simulink model "BCM2_4"  (R2021b)
settings: Solver=FixedStepDiscrete  StartTime=0.0  StopTime=1  FixedStep=0.001  RelTol=1e-3  EnableMultiTasking=on
InitFcn:
  | mbd_mpc_consistency_checks(bdroot(gcs));
model workspace (MAT data in the model file):
  CAN_rec : Simulink.Signal (value not decoded)
  CAN_transm_stat : Simulink.Signal (value not decoded)
  CAN_trm : Simulink.Signal (value not decoded)
  DITHER_CFB0 : Simulink.Parameter (value not decoded)
  DITHER_CFB1 : Simulink.Parameter (value not decoded)
  DITHER_CFB2 : Simulink.Parameter (value not decoded)
  DITHER_EN0 : Simulink.Parameter (value not decoded)
  DITHER_EN1 : Simulink.Parameter (value not decoded)
  DITHER_EN2 : Simulink.Parameter (value not decoded)
  DITHER_SIZE0 : Simulink.Parameter (value not decoded)
  DITHER_SIZE1 : Simulink.Parameter (value not decoded)
  DITHER_SIZE2 : Simulink.Parameter (value not decoded)
  DITHER_STEP0 : Simulink.Parameter (value not decoded)
  DITHER_STEP1 : Simulink.Parameter (value not decoded)
  DITHER_STEP2 : Simulink.Parameter (value not decoded)
  DITHER_SYNC0 : Simulink.Parameter (value not decoded)
  DITHER_SYNC1 : Simulink.Parameter (value not decoded)
  DITHER_SYNC2 : Simulink.Parameter (value not decoded)
  ECUMbut : Simulink.Signal (value not decoded)
  FAULTN : Simulink.Signal (value not decoded)
  FM0 : Simulink.Parameter (value not decoded)
  FM1 : Simulink.Parameter (value not decoded)
  FM2 : Simulink.Parameter (value not decoded)
  FME : Simulink.Parameter (value not decoded)
  Fsys_M : Simulink.Parameter (value not decoded)
  Fsys_N : Simulink.Parameter (value not decoded)
  Fsys_WDEN : Simulink.Parameter (value not decoded)
  Fsys_div : Simulink.Parameter (value not decoded)
  HL0 : Simulink.Parameter (value not decoded)
  HL1 : Simulink.Parameter (value not decoded)
  HL2 : Simulink.Parameter (value not decoded)
  IDIAG0 : Simulink.Parameter (value not decoded)
  IDIAG1 : Simulink.Parameter (value not decoded)
  IDIAG2 : Simulink.Parameter (value not decoded)
  Ivalve : Simulink.Signal (value not decoded)
  KI_index0 : Simulink.Parameter (value not decoded)
  KI_index1 : Simulink.Parameter (value not decoded)
  KI_index2 : Simulink.Parameter (value not decoded)
  PWM_Period0 : Simulink.Parameter (value not decoded)
  PWM_Period1 : Simulink.Parameter (value not decoded)
  PWM_Period2 : Simulink.Parameter (value not decoded)
  RESN : Simulink.Signal (value not decoded)
  SR0 : Simulink.Parameter (value not decoded)
  SR1 : Simulink.Parameter (value not decoded)
  SR2 : Simulink.Parameter (value not decoded)
  Vparam : Simulink.Signal (value not decoded)
  block_tle : Simulink.Signal (value not decoded)
  disp : Simulink.Signal (value not decoded)
  ee_adr : Simulink.Signal (value not decoded)
  ee_en_rd : Simulink.Signal (value not decoded)
  ee_en_wr : Simulink.Signal (value not decoded)
  ee_idle : Simulink.Signal (value not decoded)
  ee_read : Simulink.Signal (value not decoded)
  ee_recv : Simulink.Signal (value not decoded)
  ee_send : Simulink.Signal (value not decoded)
  in_stats : Simulink.Signal (value not decoded)
  inputs : Simulink.Signal (value not decoded)
  light : Simulink.Signal (value not decoded)
  out_drv : Simulink.Signal (value not decoded)
  out_drv_test : Simulink.Signal (value not decoded)
  out_test_en : Simulink.Signal (value not decoded)
  recv_spi2 : Simulink.Signal (value not decoded)
  ret : Simulink.Signal (value not decoded)
  spi_rcv_tle82453 : Simulink.Signal (value not decoded)
  tle82453_Ivlv : Simulink.Signal (value not decoded)
  tle82453_err : Simulink.Signal (value not decoded)
  tle82453_reset : Simulink.Signal (value not decoded)
  wtdg_CAN : Simulink.Signal (value not decoded)
symbols that are objects in the model workspace (value not decoded): CAN_rec, CAN_transm_stat, ECUMbut, inputs, Ivalve, out_drv_test, recv_spi2, ret, SR0, tle82453_Ivlv
undefined symbols (not defined in the file or in its folder): color, LQFP
libraries: simulink x68, mbd_mpc574x_ec_toolbox x50, canmsglib x42, hdlsllib x9, commutil2 x7, etargetslib x4
(part 6 of 6)

== stateflow chart BCM2_4/ecumaster12 ==
  settings: updateMethod=DISCRETE  sampleTime=0.01
  state scan_buttons [function]
    (default) -> (junction 38)
    (junction 38) -> (junction 40) : {index=1;}
    (junction 40) -> (junction 39) [order 1] : [index<13]
    (junction 39) -> (junction 46) [order 2]
    (junction 46) -> (junction 40) : {index = index + 1}
    (junction 39) -> (junction 44) [order 1] : [~ECUMbut.arr12(index) && trig(index)]{trig(index)=false}
    (junction 40) -> (junction 43) [order 2]
    (junction 44) -> (junction 46)
  state off
    scan_buttons()
    button_work()
  state button_work [function]
    note: Управление доп фарами
    note: Управление габаритами и ближним
    note: Аварийка
    note: Яркость пилота
    note: Check АКП
    note: Вентилятор пилота
    note: Таблицы ДВС
    note: Обогрев лобового стекла
    note: Электросигнал
    note: Подпирающий топливный насос
    note: Страницы -
    note: Страницы +
    note: Моргание аварийкой
    (default) -> (junction 519)
    (junction 519) -> (junction 521) [order 1] : [ECUMbut.arr12(1) && ~trig(1)]{trig(1)=true}
    (junction 521) -> (junction 530) : {light.dop=~light.dop}
    (junction 530) -> (junction 531) [order 1] : [light.dop]{ECUMbut.color12(1) = color.blue}
    (junction 519) -> (junction 599) [order 2]
    (junction 530) -> (junction 520) [order 2] : {ECUMbut.color12(1) = color.off}
    (junction 531) -> (junction 528)
    (junction 520) -> (junction 599)
    (junction 528) -> (junction 520)
    (junction 599) -> (junction 589)
    (junction 589) -> (junction 577) [order 1] : [ECUMbut.arr12(2) && ~trig(2)]{trig(2)=true}
    (junction 577) -> (junction 584) [order 1] : [cnt_light <2]{cnt_light = cnt_light + 1}
    (junction 570) -> (junction 576) [order 1] : [cnt_light==2]{light.light=true;light.beam=true;ECUMbut.color12(2) = color.blue}
    (junction 589) -> (junction 653) [order 2]
    (junction 577) -> (junction 582) [order 2]
    (junction 584) -> (junction 568)
    (junction 576) -> (junction 579)
    (junction 582) -> (junction 568) : {cnt_light=0}
    (junction 568) -> (junction 570)
    (junction 570) -> (junction 579) [order 2] : [cnt_light==1]{light.light=true;light.beam=false;ECUMbut.color12(2) = color.green}
    (junction 570) -> (junction 575) [order 3] : {light.light=false;light.beam=false;ECUMbut.color12(2) = color.off}
    (junction 579) -> (junction 575)
    (junction 575) -> (junction 653)
    (junction 653) -> (junction 514)
    (junction 514) -> (junction 553) [order 1] : [ECUMbut.arr12(3) && ~trig(3)]{trig(3)=true}
    (junction 553) -> (junction 554) : {ECUMbut.hazard=~ECUMbut.hazard}
    (junction 514) -> (junction 502) [order 2]
    (junction 554) -> (junction 555)
    (junction 555) -> (junction 502)
    (junction 502) -> (junction 516)
    (junction 516) -> (junction 546) [order 1] : [ECUMbut.arr12(4) && ~trig(4)]{trig(4)=true}
    (junction 546) -> (junction 535) : {ECUMbut.bright_pilot=~ECUMbut.bright_pilot}
    (junction 535) -> (junction 539) [order 1] : [ECUMbut.bright_pilot]{ECUMbut.color12(4) = color.bluegreen}
    (junction 516) -> (junction 560) [order 2]
    (junction 535) -> (junction 542) [order 2] : {ECUMbut.color12(4) = color.off}
    (junction 539) -> (junction 540)
    (junction 542) -> (junction 560)
    (junction 540) -> (junction 542)
    (junction 560) -> (junction 504)
    (junction 504) -> (junction 485) [order 1] : [ECUMbut.arr12(5)]{ECUMbut.color12(5) = color.orange}
    (junction 485) -> (junction 490)
    (junction 504) -> (junction 602) [order 2]
    (junction 602) -> (junction 490) [order 1] : [~ECUMbut.arr12(5)]{ECUMbut.color12(5) = color.off}
    (junction 490) -> (junction 475)
    (junction 602) -> (junction 496) [order 2]
    (junction 475) -> (junction 496)
    (junction 496) -> (junction 505)
    (junction 483) -> (junction 487) : {ECUMbut.fan=~ECUMbut.fan}
    (junction 487) -> (junction 489) [order 1] : [ECUMbut.fan]{ECUMbut.color12(6) = color.red}
    (junction 505) -> (junction 483) [order 1] : [ECUMbut.arr12(6) && ~trig(6)]{trig(6)=true}
    (junction 487) -> (junction 471) [order 2] : {ECUMbut.color12(6) = color.off}
    (junction 489) -> (junction 482)
    (junction 505) -> (junction 517) [order 2]
    (junction 471) -> (junction 517)
    (junction 482) -> (junction 471)
    (junction 517) -> (junction 499)
    (junction 499) -> (junction 615) [order 1] : [ECUMbut.arr12(7) && ~trig(7)]{trig(7)=true}
    (junction 615) -> (junction 564) : {ECUMbut.table_rom = ~ECUMbut.table_rom}
    (junction 564) -> (junction 597) [order 1] : [ECUMbut.table_rom]{ECUMbut.color12(7) = color.red}
    (junction 499) -> (junction 491) [order 2]
    (junction 564) -> (junction 592) [order 2] : {ECUMbut.color12(7) = color.off}
    (junction 597) -> (junction 593)
    (junction 592) -> (junction 491)
    (junction 593) -> (junction 592)
    (junction 491) -> (junction 498)
    (junction 498) -> (junction 618) [order 1] : [ECUMbut.arr12(8) && ~trig(8)]{trig(8)=true}
    (junction 618) -> (junction 623) : {ECUMbut.heat=~ECUMbut.heat}
    (junction 623) -> (junction 612) [order 1] : [ECUMbut.heat]{ECUMbut.color12(8) = color.green}
    (junction 498) -> (junction 493) [order 2]
    (junction 623) -> (junction 619) [order 2] : {ECUMbut.color12(8) = color.off}
    (junction 612) -> (junction 613)
    (junction 613) -> (junction 619)
    (junction 619) -> (junction 493)
    (junction 493) -> (junction 466)
    (junction 466) -> (junction 611) [order 1] : [ECUMbut.arr12(9)]{ECUMbut.color12(9) = color.orange}
    (junction 466) -> (junction 660) [order 2]
    (junction 611) -> (junction 617)
    (junction 660) -> (junction 617) [order 1] : [~ECUMbut.arr12(9)]{ECUMbut.color12(9) = color.off}
    (junction 617) -> (junction 610)
    (junction 660) -> (junction 650) [order 2]
    (junction 610) -> (junction 650)
    (junction 650) -> (junction 661)
    (junction 661) -> (junction 629) [order 1] : [ECUMbut.arr12(10) && ~trig(10)]{trig(10)=true}
    (junction 629) -> (junction 563) : {ECUMbut.pump=~ECUMbut.pump}
    (junction 563) -> (junction 608) [order 1] : [ECUMbut.pump]{ECUMbut.color12(10) = color.bluegreen}
    (junction 661) -> (junction 463) [order 2]
    (junction 563) -> (junction 594) [order 2] : {ECUMbut.color12(10) = color.off}
    (junction 608) -> (junction 625)
    (junction 625) -> (junction 594)
    (junction 594) -> (junction 463)
    (junction 463) -> (junction 465)
    (junction 465) -> (junction 621) [order 1] : [ECUMbut.arr12(11)]{ECUMbut.color12(11) = color.white}
    (junction 465) -> (junction 603) [order 2]
    (junction 621) -> (junction 646)
    (junction 603) -> (junction 646) [order 1] : [~ECUMbut.arr12(11)]{ECUMbut.color12(11) = color.off}
    (junction 646) -> (junction 642)
    (junction 603) -> (junction 666) [order 2]
    (junction 642) -> (junction 666)
    (junction 666) -> (junction 664)
    (junction 664) -> (junction 649) [order 1] : [ECUMbut.arr12(12)]{ECUMbut.color12(12) = color.white}
    (junction 664) -> (junction 657) [order 2]
    (junction 649) -> (junction 507)
    (junction 657) -> (junction 507) [order 1] : [~ECUMbut.arr12(12)]{ECUMbut.color12(12) = color.off}
    (junction 657) -> (junction 655) [order 2]
    (junction 507) -> (junction 630)
    (junction 630) -> (junction 655)
    (junction 655) -> (junction 667)
    (junction 667) -> (junction 671) [order 1] : [lamp_hazard]{ECUMbut.color12(3) = color.red}
    (junction 667) -> (junction 675) [order 2]
    (junction 671) -> (junction 678)
    (junction 675) -> (junction 678) [order 1] : [~lamp_hazard]{ECUMbut.color12(3) = color.off}
    (junction 675) -> (junction 684) [order 2]
    (junction 678) -> (junction 682)
    (junction 682) -> (junction 684)
  (default) -> off
  data: trig local boolean size=[1 12] =false; cnt_light local uint8 size=1 =uint8(0); lamp_hazard input boolean size=1; ECUMbut data_store_memory; light data_store_memory

== stateflow chart BCM2_4/поворотники ==
  settings: updateMethod=DISCRETE  sampleTime=0.1
  state blink
    state Delay
      en: i=0
      scan(true)
      du: i = i + 1
    state Delay1
      en: i=0
      scan(false)
      du: i = i + 1
    (default) -> Delay
    Delay1 -> Delay : [i>4]
    Delay -> Delay1 : [i>2]
  state scan(x) [function]
    (default) -> (junction 14)
    (junction 14) -> (junction 26) [order 1] : [left]{outL=x}
    (junction 26) -> (junction 28)
    (junction 14) -> (junction 28) [order 2]
    (junction 28) -> (junction 31) [order 1] : [right]{outR=x}
    (junction 31) -> (junction 33)
    (junction 28) -> (junction 33) [order 2]
    (junction 33) -> (junction 36) [order 1] : [hazard]{outR=x;outL=x;outH=x}
    (junction 36) -> (junction 38)
    (junction 33) -> (junction 38) [order 2]
  state start
    outL=false
    outR = false
    outH = false
  (default) -> start
  start -> blink : [left || right || hazard]
  blink -> start : [~left && ~right && ~hazard]
  data: x function_input; i local uint8 size=1; hazard input boolean size=1; left input boolean size=1; right input boolean size=1; outH output boolean size=1; outL output boolean size=1; outR output boolean size=1

== stateflow chart BCM2_4/CAN1 Transmit buf 27-43/Цвет клавиатуры 12 buf = 28/Цвет клавиатуры buf = 28/Chart ==
  (default) -> (junction 58)
  (junction 58) -> (junction 46) : {temp=0;}
  (junction 46) -> (junction 48) : {i=0;}
  (junction 48) -> (junction 57) [order 2] : {out[0] = (temp & 255);
      |  out[1] = (temp>>8) & 255;
      |  out[2] = (temp>>16)  & 255;
      |  out[3] = (temp>>24)  & 255;}
  (junction 48) -> (junction 47) [order 1] : [i<12]
  (junction 50) -> (junction 48)
  (junction 47) -> (junction 49) : {temp = temp | (input[i] & 1) << (0+i);
      | temp = temp | ((input[i] & 2)>>1) << (12 + i);
      | temp = temp | ((input[i] & 4)>>2) << (24 + i);}
  (junction 49) -> (junction 50) : {i++;}
  data: i local uint8 size=1 =uint8(0); input input uint8 size=12; temp local double size=1; out output uint8 size=8

== stateflow chart BCM2_4/CAN1 Transmit buf 27-43/подсветка клавиатуры buf = 29/подсветка клавиатуры buf = 29/Chart ==
  state backlight_bright
    en:
    out(1) = 0x2F
    out(2) = 3
    out(3) = 0x20
    out(4) = 2
    out(5) = 0x00 % level
  state key_bright1
    en:
    out(1) = 0x2F
    out(2) = 3
    out(3) = 0x20
    out(4) = 1
    out(5) = 0x0F %level
  note: Яркость клавиш при вкл подсветки клавиш
  state backlight_color1
    en:
    out(1) = 0x2F
    out(2) = 3
    out(3) = 0x20
    out(4) = 4
    out(5) = 9
  note: red(1)
      | green(2)
      | blue(3)
      | yellow(4)
      | bluegreen(5)
      | purple(6)
      | white(7)
      | orange(8)
      | yel_green(9)
  state key_bright
    en:
    out(1) = 0x2F
    out(2) = 3
    out(3) = 0x20
    out(4) = 1
    out(5) = 0x30 %level
  state backlight_bright1
    en:
    out(1) = 0x2F
    out(2) = 3
    out(3) = 0x20
    out(4) = 2
    out(5) = 0x04 % level
  note: Яркость подсветки
  note: Яркость клавиш
  (default) -> backlight_bright
  key_bright1 -> backlight_bright : [~ECUMbut.bright_pilot]
  backlight_bright -> key_bright
  backlight_color1 -> key_bright1
  backlight_bright1 -> backlight_color1
  key_bright -> backlight_bright1 : [ECUMbut.bright_pilot]
  data: out output uint8 size=8; ECUMbut data_store_memory

== stateflow chart BCM2_4/retarder ==
  settings: updateMethod=DISCRETE  sampleTime=0.1
  state Diagnostic
    en:
    Ivalve(1)=0
    Ivalve(2)=0
  state work
    state ret_off
      Ivalve(1)=0
      Ivalve(2)=0
    state ret_on
      state ret_on
        ret.M = uint16(ret.stepM(ret.step) * 4000)
        Ivalve(1)=450
      state ret_stdby
        Ivalve(1)=0
        Ivalve(2)=0
      state table
      (default) -> ret_stdby
      ret_stdby -> work.ret_on.ret_on : [Vparam.BrakePos > brk_lvl]
      work.ret_on.ret_on -> ret_stdby [order 1] : [Vparam.BrakePos < (brk_lvl - 2)]
      work.ret_on.ret_on -> table [order 2]
      table -> work.ret_on.ret_on
    state temp_protect
      Ivalve(1)=0
      Ivalve(2)=0
    state diable_pedal
      Ivalve(1)=0
      Ivalve(2)=0
    (default) -> ret_off
    work.ret_on -> ret_off [order 1] : [~ret.ret_en]
    ret_off -> work.ret_on : [ret.ret_en]
    work.ret_on -> temp_protect [order 2] : [ret.RetTemp > 145]
    temp_protect -> work.ret_on : [ret.RetTemp < 120]
    work.ret_on -> diable_pedal [order 3] : [Vparam.PedalPos > 3]
    diable_pedal -> work.ret_on : [Vparam.PedalPos < 1]
  (default) -> Diagnostic
  Diagnostic -> work : [diag == false]
  work -> Diagnostic : [diag == true]
  data: sf_internal_action_state_placeholder_data local double size=1 =0; ret data_store_memory; Vparam data_store_memory; brk_lvl constant uint8 =5; Ivalve data_store_memory; temp_protect output boolean; diable_pedal output boolean; diag input boolean

== stateflow chart BCM2_4/подогрев стекла ==
  settings: updateMethod=DISCRETE  sampleTime=1
  state off
    out = false
  state on
    state on
      en: i=1
      out=true
      du: i = i + 1
    state off
      en: i=1
      out=false
      du: i = i + 1
    (default) -> on.on
    on.off -> on.on : [i>=heat_off * 60]
    on.on -> on.off : [i>=heat_on * 60]
  (default) -> off
  off -> on : [heat]
  on -> off : [~heat]{out=false}
  data: out output boolean size=1; i local; heat input boolean size=1; heat_on parameter; heat_off parameter

== stateflow chart BCM2_4/CAN EEPROM R//W ==
  state ee_wr
    ee_adr = CAN_rec.ee_adr
    ee_send = CAN_rec.ee_data
    % записываем в eeprom
  state x = ee_idl [function]
    (default) -> (junction 28)
    (junction 28) -> (junction 29) [order 1] : [~ee_idle && ~ee_en_rd && ~ee_en_wr]
    (junction 29) -> (junction 31)
    (junction 28) -> (junction 30) [order 2] : {x=true}
    (junction 31) -> (junction 30) : {x = false}
  state ee_idle
    % свободна ли EEPROM?
  state Start
  state ee_idle1
  state ee_idle2
  state ready
    en:
    CAN_trm.ee_adr=CAN_rec.ee_adr;
    CAN_trm.ee_cmd = CAN_rec.ee_cmd;
    CAN_trm.ee_data = ee_read;
    ex: ee_en_rd = false % выключаем чтение из еепром
    CAN_rec.ee_rec_stat = false;
    CAN_trm.ee_en_trm = true;
  state ee_rd
    % запускаем чтение с еепром
  ee_idle -> ee_wr : [~ee_idle && ~ee_en_rd && ~ee_en_wr]{ee_en_wr = true}
  (junction 3) -> ee_idle [order 2] : [CAN_rec.ee_cmd == CMD_WRITE]
  ee_wr -> (junction 66) : [~ee_idle]% ждем окончания записи
      | {ee_en_wr = false}% отключаем запись eeprom
  (default) -> Start
  ee_idle2 -> ee_idle1 [order 2]
  Start -> (junction 3) : [CAN_rec.ee_rec_stat]
  (junction 3) -> ee_idle1 [order 1] : [CAN_rec.ee_cmd == CMD_READ]
  (junction 3) -> (junction 48) [order 3]
  ee_idle1 -> ee_idle2 : [~ee_idl]
      | % ждем готовность еепром
  ee_idle2 -> ee_rd [order 1] : [~ee_idl]{ee_adr = CAN_rec.ee_adr; ee_en_rd = true;}
  (junction 48) -> Start
  ee_rd -> ready : [~ee_idle] % дожидаемся конца чтения
  ready -> Start
  (junction 66) -> ready
  data: x function_output; CAN_rec data_store_memory; CMD_READ constant double =3; CMD_WRITE constant double =6; ee_idle data_store_memory; ee_adr data_store_memory; ee_en_rd data_store_memory; ee_read data_store_memory; ee_en_wr data_store_memory; CAN_trm data_store_memory; ee_send data_store_memory

== stateflow chart BCM2_4/управление страницами и яркостью мониторов/eeprom страницы ==
  state x = ee_idl [function]
    (default) -> (junction 16)
    (junction 16) -> (junction 17) [order 1] : [~ee_idle && ~ee_en_rd && ~ee_en_wr]
    (junction 17) -> (junction 19)
    (junction 16) -> (junction 18) [order 2] : {x=true}
    (junction 19) -> (junction 18) : {x = false}
  state ee_idle1
  state ee_idle2
  state ee_rd
    % запускаем чтение с еепром
  state ready
    en:  disp.meh_page = uint8(bitand(ee_read,255))
    disp.pilot_page = uint8(bitshift(ee_read, -8))
    ex: ee_en_rd = false % выключаем чтение из еепром
  state idle
  state wait_write_ee
  state ee_idle
    % свободна ли EEPROM?
  state ee_wr
    ee_adr = adres_page
    ee_send = 0
    ee_send = bitor(ee_send,uint16(disp.meh_page))
    ee_send = bitor(ee_send,bitshift(uint16(disp.pilot_page),8))
    % записываем в eeprom
  (default) -> ee_idle1
  ee_idle2 -> ee_idle1 [order 2]
  ee_idle1 -> ee_idle2 : [~ee_idl]
      | % ждем готовность еепром
  ee_idle2 -> ee_rd [order 1] : [~ee_idl]{ee_adr = adres_page; ee_en_rd = true;}
  ee_rd -> ready : [~ee_idle] % дожидаемся конца чтения
  ready -> (junction 48)
  (junction 48) -> (junction 49) [order 1] : [disp.meh_page>disp.meh_max_page]{disp.meh_page = 1}
  (junction 49) -> (junction 51)
  (junction 48) -> (junction 51) [order 2]
  (junction 51) -> (junction 54) [order 1] : [disp.pilot_page>disp.pilot_max_page]{disp.pilot_page = 1}
  (junction 51) -> idle [order 2]
  (junction 54) -> idle
  idle -> ee_idle : [write_ee]
  wait_write_ee -> idle : [~write_ee]
  ee_wr -> wait_write_ee : [~ee_idle]% ждем окончания записи
      | {ee_en_wr = false}% отключаем запись eeprom
  ee_idle -> ee_wr : [~ee_idle && ~ee_en_rd && ~ee_en_wr]{ee_en_wr = true}
  data: x function_output; ee_idle data_store_memory; ee_read data_store_memory; ee_adr data_store_memory; ee_en_rd data_store_memory; disp data_store_memory; adres_page constant uint8 =uint8(126); ee_en_wr data_store_memory; write_ee input; ee_send data_store_memory

== stateflow chart BCM2_4/Степы ретардера/eeprom степы ретардера ==
  state x = ee_idl [function]
    (default) -> (junction 16)
    (junction 16) -> (junction 17) [order 1] : [~ee_idle && ~ee_en_rd && ~ee_en_wr]
    (junction 17) -> (junction 19)
    (junction 16) -> (junction 18) [order 2] : {x=true}
    (junction 19) -> (junction 18) : {x = false}
  state ee_idle1
  state ee_idle2
  state ee_rd
    % запускаем чтение с еепром
  state ready
    en:  ret.step_brk = uint8(bitand(ee_read,255))
    ret.step = uint8(bitshift(ee_read, -8))
    ex: ee_en_rd = false % выключаем чтение из еепром
  state idle
  state wait_write_ee
  state ee_idle
    % свободна ли EEPROM?
  state ee_wr
    ee_adr = adres_page
    ee_send = 0
    ee_send = bitor(ee_send,uint16(ret.step_brk))
    ee_send = bitor(ee_send,bitshift(uint16(ret.step),8))
    % записываем в eeprom
  (default) -> ee_idle1
  ee_idle2 -> ee_idle1 [order 2]
  ee_idle1 -> ee_idle2 : [~ee_idl]
      | % ждем готовность еепром
  ee_idle2 -> ee_rd [order 1] : [~ee_idl]{ee_adr = adres_page; ee_en_rd = true;}
  ee_rd -> ready : [~ee_idle] % дожидаемся конца чтения
  ready -> idle
  idle -> idle [order 3] : [ret.step_brk> step_brk_max]{ret.step_brk = 1}
  idle -> idle [order 2] : [ret.step>step_max]{ret.step = 1}
  idle -> ee_idle [order 1] : [write_ee]
  wait_write_ee -> idle : [~write_ee]
  ee_wr -> wait_write_ee : [~ee_idle]% ждем окончания записи
      | {ee_en_wr = false}% отключаем запись eeprom
  ee_idle -> ee_wr : [~ee_idle && ~ee_en_rd && ~ee_en_wr]{ee_en_wr = true}
  data: x function_output; ee_idle data_store_memory; ee_read data_store_memory; ee_adr data_store_memory; ee_en_rd data_store_memory; adres_page constant uint8 =uint8(125); ee_en_wr data_store_memory; write_ee input; ee_send data_store_memory; step_brk_max input; step_max input; ret data_store_memory

== stateflow chart BCM2_4/Расход топлива/Расход топлива ==
  settings: updateMethod=DISCRETE  sampleTime=0.01
  state x = ee_idl [function]
    (default) -> (junction 33)
    (junction 33) -> (junction 34) [order 1] : [~ee_idle && ~ee_en_rd && ~ee_en_wr]
    (junction 34) -> (junction 36)
    (junction 33) -> (junction 35) [order 2] : {x=true}
    (junction 36) -> (junction 35) : {x = false}
  state Read EEPROM [group]
    state ee_idle1
    state ee_idle2
    state ee_rd
      % запускаем чтение с еепром
    (default) -> Read.ee_idle1
    (junction 131) -> Read.ee_idle1 [order 1] : [i<2]
    (junction 129) -> (junction 131) : {ee_en_rd = false}
    Read.ee_idle1 -> ee_idle2 : [~ee_idl]
        | % ждем готовность еепром
    ee_idle2 -> Read.ee_idle1 [order 2]
    ee_idle2 -> (junction 98) [order 1]
    (junction 98) -> (junction 99) [order 1] : [~ee_idl && i==0]
        | {ee_adr = adres_distH; ee_en_rd = true;}
    (junction 98) -> (junction 101) [order 2]
    (junction 99) -> (junction 103)
    (junction 101) -> (junction 103) [order 1] : [~ee_idl && i==1]
        | {ee_adr = adres_distL; ee_en_rd = true;}
    (junction 101) -> (junction 107) [order 2]
    (junction 103) -> (junction 109)
    (junction 107) -> (junction 109) : [~ee_idl && i==2]
        | {ee_adr = adres_fuel; ee_en_rd = true;}
    (junction 109) -> ee_rd
    ee_rd -> (junction 114) : [~ee_idle]
        | % дожидаемся конца чтения
    (junction 114) -> (junction 115) [order 1] : [i==0]{distH = ee_read}
    (junction 114) -> (junction 119) [order 2]
    (junction 115) -> (junction 121)
    (junction 119) -> (junction 121) [order 1] : [i==1]{distL = ee_read}
    (junction 119) -> (junction 123) [order 2]
    (junction 121) -> (junction 125)
    (junction 123) -> (junction 125) : [i==2]{Temp_fuel = ee_read}
    (junction 125) -> (junction 129) : {i = i + 1}
  state Write EEPROM [group]
    state init_write
      Temp_dist = dist;
      Temp_fuel = fuel;
      i=0;
      distL = uint16(bitand(Temp_dist,65535))
      distH = uint16(bitshift(Temp_dist, -16))
    state ee_idle1
      % свободна ли EEPROM?
    state ee_wr2
      % записываем в eeprom
    state wait_trip
    init_write -> Write.ee_idle1
    (junction 169) -> Write.ee_idle1 [order 1] : [i<2]
    Write.ee_idle1 -> (junction 152) : [~ee_idle && ~ee_en_rd && ~ee_en_wr]{ee_en_wr = true}
    (junction 152) -> (junction 153) [order 1] : [i==0]{ee_adr = adres_distH; ee_send = distH;}
    (junction 152) -> (junction 156) [order 2]
    (junction 153) -> (junction 158)
    (junction 156) -> (junction 158) [order 1] : [i==1]{ee_adr = adres_distL; ee_send = distL;}
    (junction 158) -> (junction 162)
    (junction 156) -> (junction 160) [order 2]
    (junction 160) -> (junction 162) : [i==2]{ee_adr = adres_fuel; ee_send = Temp_fuel;}
    (junction 162) -> ee_wr2
    ee_wr2 -> (junction 169) : [~ee_idle]% ждем окончания записи
        | {ee_en_wr = false; i = i + 1;}
    (junction 169) -> wait_trip [order 2]
  state wait
    i = i + 1
  (junction 131) -> (junction 179) [order 2] : {Temp_dist = bitor(Temp_dist,uint32(distL));
      | Temp_dist = bitor(Temp_dist,bitshift(uint32(distH),16)); }
  (junction 179) -> wait
  wait -> init_write [order 1] : [trip]
  (junction 26) -> wait : {i=0}
  (junction 24) -> (junction 26)
  (junction 176) -> wait
  wait -> (junction 20) [order 2] : [i>100]
  (junction 20) -> (junction 22)
  (junction 22) -> (junction 24) : {r=((double(Temp_fuel - fuel))/(double(dist-Temp_dist)))*100}
  wait_trip -> (junction 176) : [~trip]
  data: x function_output; Temp_dist local uint32 =uint32(0); Temp_fuel local uint16 =uint16(0); trip input boolean; fuel input uint16; i local uint8 =uint8(0); r output double =0; dist input uint32; adres_distH constant uint8 =uint8(124); ee_en_rd data_store_memory; ee_adr data_store_memory; adres_fuel constant uint8 =uint8(122); ee_idle data_store_memory; ee_read data_store_memory; ee_en_wr data_store_memory; ee_send data_store_memory; adres_distL constant uint8 =uint8(123); distH local uint16; distL local uint16

== stateflow chart BCM2_4/перекачка ==
  settings: updateMethod=DISCRETE  sampleTime=0.1
  state start
  state delay_work
    en: i=0;
    du:
    i = i + 1;
    ex:
    pump1 = false;
    pump2 = false;
  note: Опустошение баков
  state delay_meas
    en: i=0;
    du:
    i = i + 1;
    ex:
  state delay_work1
    en: i=0;
    du:
    i = i + 1;
    ex:
    pump1 = false;
    pump2 = false;
  state delay_meas1
    en: i=0;
    du:
    i = i + 1;
    ex:
  (junction 83) -> (junction 85)
  start -> (junction 83) [order 5] : [tank2>1 && pump_trig2]{pump_trig2 = false}
  (junction 85) -> (junction 87)
  (junction 81) -> (junction 87)
  start -> (junction 81) [order 4] : [tank1>1 && pump_trig1]{pump_trig1 = false}
  (junction 87) -> start
  (junction 26) -> (junction 46) [order 1] : [err2]{err2 = err2 - 1}
  (junction 25) -> (junction 26) [order 1] : [err1< 3 && tank1>tank2 && tank1>0]{pump1=true;pri=1;}
  (default) -> start
  (junction 26) -> (junction 43) [order 2]
  (junction 46) -> (junction 43)
  start -> (junction 25) [order 1] : [tank3<160]
  (junction 25) -> (junction 28) [order 2] : [err2< 3 && tank2>0]{pump2 = true;pri=2;}
  (junction 25) -> (junction 69) [order 3]
  (junction 39) -> (junction 25) [order 1] : [tank3<180]
  (junction 43) -> delay_work : {temp = tank3}
  (junction 69) -> start
  (junction 49) -> (junction 43)
  delay_meas1 -> start : [i>=150]% время паузы перед замером топлива секунды*10
  start -> delay_work1 [order 3] : [tank3 < 40 && tank2<1 && ~pump_trig2]{pump1=true; pump_trig2=true;}
  start -> delay_work1 [order 2] : [tank3 < 40 && tank1<1 && ~pump_trig1]{pump1=true; pump_trig1=true;}
  (junction 39) -> start [order 2]
  (junction 28) -> (junction 49) [order 2]
  (junction 48) -> (junction 49)
  delay_work -> delay_meas : [i>=200]% время работы насосов секунды*10
  (junction 28) -> (junction 48) [order 1] : [err1]{err1 = err1 - 1}
  (junction 58) -> (junction 61) [order 1] : [pri==1]{err1 = err1 + 1}
  (junction 61) -> (junction 63)
  (junction 58) -> (junction 63) [order 2] : [pri==2]{err2 = err2 + 1}
  (junction 57) -> (junction 58) [order 1] : [tank3<=temp]
  (junction 63) -> (junction 66)
  (junction 66) -> (junction 39)
  (junction 57) -> (junction 66) [order 2]
  delay_meas -> (junction 57) : [i>=150]% время паузы перед замером топлива секунды*10
  delay_work1 -> delay_meas1 : [i>=300]% время работы насосов секунды*10
  data: tank1 input; tank2 input; tank3 input; pump1 output =false; pump2 output =false; i local; err1 local size=1 =0; err2 local size=1 =0; pri local; temp local; pump_trig1 local; pump_trig2 local

== stateflow chart BCM2_4/CAN1 Transmit buf 27-43/подсветка клавиатуры buf = 31/подсветка клавиатуры buf = 31/Chart ==
  state backlight_bright
    en:
    out(1) = 0x2F
    out(2) = 3
    out(3) = 0x20
    out(4) = 2
    out(5) = 0x00 % level
  state key_bright1
    en:
    out(1) = 0x2F
    out(2) = 3
    out(3) = 0x20
    out(4) = 1
    out(5) = 0x0F %level
  note: Яркость клавиш при вкл подсветки клавиш
  state backlight_color1
    en:
    out(1) = 0x2F
    out(2) = 3
    out(3) = 0x20
    out(4) = 4
    out(5) = 9
  note: red(1)
      | green(2)
      | blue(3)
      | yellow(4)
      | bluegreen(5)
      | purple(6)
      | white(7)
      | orange(8)
      | yel_green(9)
  state key_bright
    en:
    out(1) = 0x2F
    out(2) = 3
    out(3) = 0x20
    out(4) = 1
    out(5) = 0x30 %level
  state backlight_bright1
    en:
    out(1) = 0x2F
    out(2) = 3
    out(3) = 0x20
    out(4) = 2
    out(5) = 0x04 % level
  note: Яркость подсветки
  note: Яркость клавиш
  (default) -> backlight_bright
  key_bright1 -> backlight_bright : [~ECUMbut.bright_pilot]
  backlight_bright -> key_bright
  backlight_color1 -> key_bright1
  backlight_bright1 -> backlight_color1
  key_bright -> backlight_bright1 : [ECUMbut.bright_pilot]
  data: out output uint8 size=8; ECUMbut data_store_memory

== stateflow chart BCM2_4/Управление с клавиатуры ECUMASTER/Chart1 ==
  settings: updateMethod=DISCRETE  sampleTime=0.01
  state Motor_pilot [parallel]
    settings: executionOrder=1
    state start
    state stop
      en: i=0
      PM_up = true;
      du: i = i + 1
      %включаем мотор вверх
    state avto
    state auto_stop
      PM_up = false
      PM_dn = false
    state stop1
      en: i=0
      PM_dn = true;
      du: i = i + 1
      %включаем мотор вверх
    (default) -> Motor_pilot.start
    Motor_pilot.start -> Motor_pilot.stop [order 1] : [ButP_up]
        | % если кнопка нажата
    Motor_pilot.stop -> Motor_pilot.avto [order 2] : [~ButP_up]
    Motor_pilot.stop -> Motor_pilot.auto_stop [order 1] : [i>20 && ~ButP_up]
    Motor_pilot.stop -> Motor_pilot.auto_stop [order 3] : [I_MP>7]
    Motor_pilot.auto_stop -> Motor_pilot.start : [~ButP_up && ~ButP_dn]
    Motor_pilot.avto -> Motor_pilot.auto_stop [order 1] : [I_MP>7]
    Motor_pilot.avto -> Motor_pilot.auto_stop [order 2] : [ButP_dn || ButP_up]
    Motor_pilot.stop1 -> Motor_pilot.auto_stop [order 1] : [i>20 && ~ButP_dn]
    Motor_pilot.stop1 -> Motor_pilot.auto_stop [order 3] : [I_MP>7]
    Motor_pilot.start -> Motor_pilot.stop1 [order 2] : [ButP_dn]
        | % если кнопка нажата
    Motor_pilot.stop1 -> Motor_pilot.avto [order 2] : [~ButP_dn]
  state Motor_meh [parallel]
    settings: executionOrder=2
    state start
    state stop
      en: i2=0
      MM_up = true;
      du: i2 = i2 + 1
      %включаем мотор вверх
    state avto
    state auto_stop
      MM_up = false
      MM_dn = false
    state stop1
      en: i2=0
      MM_dn = true;
      du: i2 = i2 + 1
      %включаем мотор вверх
    (default) -> Motor_meh.start
    Motor_meh.start -> Motor_meh.stop [order 1] : [ButM_up]
        | % если кнопка нажата
    Motor_meh.stop -> Motor_meh.avto [order 2] : [~ButM_up]
    Motor_meh.stop -> Motor_meh.auto_stop [order 1] : [i2>20 && ~ButM_up]
    Motor_meh.stop -> Motor_meh.auto_stop [order 3] : [I_MM>7]
    Motor_meh.auto_stop -> Motor_meh.start : [~ButM_up && ~ButM_dn]
    Motor_meh.avto -> Motor_meh.auto_stop [order 1] : [I_MM>7]
    Motor_meh.avto -> Motor_meh.auto_stop [order 2] : [ButM_dn || ButM_up]
    Motor_meh.stop1 -> Motor_meh.auto_stop [order 1] : [i2>20 && ~ButM_dn]
    Motor_meh.stop1 -> Motor_meh.auto_stop [order 3] : [I_MM>7]
    Motor_meh.stop1 -> Motor_meh.avto [order 2] : [~ButM_dn]
    Motor_meh.start -> Motor_meh.stop1 [order 2] : [ButM_dn]
        | % если кнопка нажата
  data: ButP_up input boolean; ButP_dn input boolean; ButM_up input boolean; ButM_dn input boolean; PM_up output boolean =false; PM_dn output boolean =false; MM_up output boolean =false; MM_dn output boolean =false; I_MP input; i local =0; i2 local; I_MM input

== stateflow chart BCM2_4/CAN WATCHDOG/WATCHDOG SCAN ==
  settings: updateMethod=DISCRETE  sampleTime=0.1
  (default) -> (junction 121)
  (junction 121) -> (junction 100) [order 1] : [wtdg_CAN.id195<20]{wtdg_CAN.id195 = wtdg_CAN.id195 + 1}
  (junction 163) -> (junction 165)
  (junction 165) -> (junction 167) [order 1] : [wtdg_CAN.VD<20]{wtdg_CAN.VD = wtdg_CAN.VD + 1}
  (junction 167) -> (junction 169)
  (junction 100) -> (junction 104)
  (junction 121) -> (junction 104) [order 2] : {id195}
  (junction 161) -> (junction 163)
  (junction 165) -> (junction 169) [order 2] : {VD}
  (junction 104) -> (junction 103) [order 1] : [wtdg_CAN.id192<20]{wtdg_CAN.id192 = wtdg_CAN.id192 + 1}
  (junction 169) -> (junction 173) [order 1] : [wtdg_CAN.FuelTank<20]{wtdg_CAN.FuelTank = wtdg_CAN.FuelTank + 1}
  (junction 173) -> (junction 175)
  (junction 103) -> (junction 107)
  (junction 104) -> (junction 107) [order 2] : {id192}
  (junction 169) -> (junction 175) [order 2] : {FuelTank}
  (junction 107) -> (junction 113) [order 1] : [wtdg_CAN.CCVS1_00<20]{wtdg_CAN.CCVS1_00 = wtdg_CAN.CCVS1_00 + 1}
  (junction 175) -> (junction 179) [order 1] : [wtdg_CAN.max_page_pilot<20]{wtdg_CAN.max_page_pilot = wtdg_CAN.max_page_pilot + 1}
  (junction 179) -> (junction 181)
  (junction 113) -> (junction 106)
  (junction 107) -> (junction 106) [order 2] : {CCVS1_00}
  (junction 175) -> (junction 181) [order 2] : {max_page_pilot}
  (junction 106) -> (junction 108) [order 1] : [wtdg_CAN.RF<20]{wtdg_CAN.RF = wtdg_CAN.RF + 1}
  (junction 181) -> (junction 185) [order 1] : [wtdg_CAN.max_page_meh<20]{wtdg_CAN.max_page_meh = wtdg_CAN.max_page_meh + 1}
  (junction 185) -> (junction 187)
  (junction 108) -> (junction 120)
  (junction 106) -> (junction 120) [order 2] : {RF}
  (junction 181) -> (junction 187) [order 2] : {max_page_meh}
  (junction 120) -> (junction 131) [order 1] : [wtdg_CAN.EBC1<20]{wtdg_CAN.EBC1 = wtdg_CAN.EBC1 + 1}
  (junction 187) -> (junction 191) [order 1] : [wtdg_CAN.w18F0010B<20]{wtdg_CAN.w18F0010B = wtdg_CAN.w18F0010B + 1}
  (junction 191) -> (junction 193)
  (junction 131) -> (junction 124)
  (junction 120) -> (junction 124) [order 2] : {EBC1}
  (junction 187) -> (junction 193) [order 2] : {w18F0010B}
  (junction 124) -> (junction 117) [order 1] : [wtdg_CAN.EEC1_400<20]{wtdg_CAN.EEC1_400 = wtdg_CAN.EEC1_400 + 1}
  (junction 193) -> (junction 197) [order 1] : [wtdg_CAN.w18FEAD0B<20]{wtdg_CAN.w18FEAD0B = wtdg_CAN.w18FEAD0B + 1}
  (junction 197) -> (junction 199)
  (junction 117) -> (junction 138)
  (junction 124) -> (junction 138) [order 2] : {EEC1_400}
  (junction 193) -> (junction 199) [order 2] : {w18FEAD0B}
  (junction 138) -> (junction 125) [order 1] : [wtdg_CAN.EEC1_300<20]{wtdg_CAN.EEC1_300 = wtdg_CAN.EEC1_300 + 1}
  (junction 199) -> (junction 203) [order 1] : [wtdg_CAN.w18FEEA2F<20]{wtdg_CAN.w18FEEA2F = wtdg_CAN.w18FEEA2F + 1}
  (junction 203) -> (junction 205)
  (junction 125) -> (junction 118)
  (junction 138) -> (junction 118) [order 2] : {EEC1_300}
  (junction 199) -> (junction 205) [order 2] : {w18FEEA2F}
  (junction 118) -> (junction 137) [order 1] : [wtdg_CAN.ETC1<20]{wtdg_CAN.ETC1 = wtdg_CAN.ETC1 + 1}
  (junction 137) -> (junction 139)
  (junction 118) -> (junction 139) [order 2] : {ETC1}
  (junction 139) -> (junction 133) [order 1] : [wtdg_CAN.ee_wr<20]{wtdg_CAN.ee_wr = wtdg_CAN.ee_wr + 1}
  (junction 133) -> (junction 128)
  (junction 139) -> (junction 128) [order 2] : {ee_wr}
  (junction 128) -> (junction 155) [order 1] : [wtdg_CAN.id101<20]{wtdg_CAN.id101 = wtdg_CAN.id101 + 1}
  (junction 155) -> (junction 157)
  (junction 128) -> (junction 157) [order 2] : {id101}
  (junction 157) -> (junction 161)
  data: wtdg_CAN data_store_memory
  events: ee_wr output FUNCTION_CALL_EVENT; id192 output FUNCTION_CALL_EVENT; id195 output FUNCTION_CALL_EVENT; CCVS1_00 output FUNCTION_CALL_EVENT; EBC1 output FUNCTION_CALL_EVENT; EEC1_300 output FUNCTION_CALL_EVENT; EEC1_400 output FUNCTION_CALL_EVENT; ETC1 output FUNCTION_CALL_EVENT; RF output FUNCTION_CALL_EVENT; id101 output FUNCTION_CALL_EVENT; VD output FUNCTION_CALL_EVENT; FuelTank output FUNCTION_CALL_EVENT; max_page_pilot output FUNCTION_CALL_EVENT; max_page_meh output FUNCTION_CALL_EVENT; w18F0010B output FUNCTION_CALL_EVENT; w18FEAD0B output FUNCTION_CALL_EVENT; w18FEEA2F output FUNCTION_CALL_EVENT

== stateflow chart BCM2_4/Drivers/Remote mc33978 ==
  state cinfig_inputs
    bool_conf1 = logical([in_bl8,in_bl7,in_bl6,in_bl5,in_bl4,in_bl3,in_bl2,in_bl1])
    bool_conf2 = logical([in_bl16,in_bl15,in_bl14,in_bl13,in_bl12,in_bl11,in_bl10,in_bl9])
    conf1 = uint8(bi2de(bool_conf1,'left-msb'))
    conf2 = uint8(bi2de(bool_conf2,'left-msb'))
    out_data =[ 0X03, 0X00, 0X08, conf1,0X03, 0X00, 0X08, conf2]
    send_spi
  state cinfig_inputs1
    out_data =[ 0X05, 0X00, 0X00, 0X00,0X05, 0X00, 0X00, 0X00]
    send_spi
  state cinfig_inputs2
    out_data =[ 0X07, 0X00, 0X00, 0X00,0X07, 0X00, 0X00, 0X00]
    send_spi
  state cinfig_inputs3
    out_data =[ 0X09, 0X00, 0X00, 0X00,0X09, 0X00, 0X00, 0X00]
    send_spi
  state cinfig_inputs4
    out_data =[ 0X0B, 0X00, 0X00, 0X00,0X0B, 0X00, 0X00, 0X00]
    send_spi
  state cinfig_inputs5
    out_data =[ 0X0D, 0X00, 0X00, 0X00,0X0D, 0X00, 0X00, 0X00]
    send_spi
  state cinfig_inputs6
    out_data =[ 0X35, 0XFF, 0XFF, 0XFF,0X35, 0XFF, 0XFF, 0XFF]
    send_spi
  state delay
    en: i=0;
    du: i = i + 1;
  state transmit
    out_data =[ 0X3E, 0XC0, 0X00, 0X00,0X3E, 0XC0, 0X00, 0X00]
    send_spi
  state transmit1
    out_data =[ 0X42, 0X00, 0X00, 0X00,0X42, 0X00, 0X00, 0X00]
    send_spi
  (default) -> cinfig_inputs
  cinfig_inputs -> cinfig_inputs1
  cinfig_inputs1 -> cinfig_inputs2
  cinfig_inputs2 -> cinfig_inputs3
  cinfig_inputs3 -> cinfig_inputs4
  cinfig_inputs4 -> cinfig_inputs5
  cinfig_inputs5 -> cinfig_inputs6
  cinfig_inputs6 -> delay
  transmit1 -> delay
  delay -> transmit : [i>=10]
  transmit -> transmit1
  data: i local; out_data output uint8 size=[1 8]; bool_conf1 local boolean size=[1 8] =logical([0 0 0 0 0 0 0 0]); bool_conf2 local boolean size=[1 8] =logical([0 0 0 0 0 0 0 0]); conf1 local uint8 size=1 =uint8(0); conf2 local uint8 size=1 =uint8(0); in_bl1 parameter; in_bl2 parameter; in_bl3 parameter; in_bl4 parameter; in_bl5 parameter; in_bl6 parameter; in_bl7 parameter; in_bl8 parameter; in_bl10 parameter; in_bl11 parameter; in_bl12 parameter; in_bl13 parameter; in_bl14 parameter; in_bl15 parameter; in_bl16 parameter; in_bl9 parameter
  events: send_spi output FUNCTION_CALL_EVENT

== stateflow chart BCM2_4/управление лепестками/Remote stab ==
  settings: updateMethod=DISCRETE  sampleTime=0.01
  state ee_idle1
  state ee_idle2
  state ee_rd
    % запускаем чтение с еепром
  state int2bit [function]
    (default) -> (junction 203)
    (junction 203) -> (junction 208) [order 1] : [bitand(ee_read,1)]{temp_fr=true}
    (junction 208) -> (junction 210)
    (junction 203) -> (junction 210) [order 2] : {temp_fr=false}
    (junction 210) -> (junction 213) [order 1] : [bitand(ee_read,2) == 2]{temp_rr=true}
    (junction 213) -> (junction 215)
    (junction 210) -> (junction 215) [order 2] : {temp_rr=false}
    (junction 215) -> (junction 257)
    (junction 257) -> (junction 259) [order 1] : [bitand(ee_read,2) == 4]{temp_ret=true}
    (junction 259) -> (junction 261)
    (junction 257) -> (junction 261) [order 2] : {temp_ret = false}
  state x = ee_idl [function]
    (default) -> (junction 184)
    (junction 184) -> (junction 187) [order 1] : [~ee_idle && ~ee_en_rd && ~ee_en_wr]
    (junction 187) -> (junction 191)
    (junction 184) -> (junction 189) [order 2] : {x=true}
    (junction 191) -> (junction 189) : {x = false}
  state ee_rd1
    en: int2bit() % конвертируем число в биты
    rele_rr_stab = temp_rr
    rele_fr_stab = temp_fr & temp_rr
    rele_ret=temp_ret
    ex: ee_en_rd = false % выключаем чтение из еепром
  state wait
    % опрос лепестков
  state ee_wr_off
    en:
    ee_en_wr = false
    % отключаем запись eeprom
  state ee_wr
    en:
    ee_adr = adres_stab
    ee_send = 0
    ee_send = bitor(ee_send,uint16(temp_fr))
    ee_send = bitor(ee_send,bitshift(uint16(temp_rr),1))
    ee_send = bitor(ee_send,bitshift(uint16(temp_ret),3))
    ee_en_wr = true
    % записываем в eeprom
  state ee_idle
    res = ee_idl
    % свободна ли EEPROM?
  state Beep1
    state Delay
      en: i=0
      zummer=true;
      du: i = i + 1
    state Delay1
      en: i=0
      zummer=false;
      du: i = i + 1
    (default) -> Delay
    Delay1 -> Delay : [i2>0 && i > 5]
    Delay -> Delay1 : [i>10]{ i2 = i2 - 1;}
  (default) -> ee_idle1
  ee_idle2 -> ee_idle1 [order 2]
  ee_idle1 -> ee_idle2 : [~ee_idl] % ждем готовность еепром
  ee_idle2 -> ee_rd [order 1] : [~ee_idl]{ee_adr = adres_stab;ee_en_rd = true;}
  ee_rd -> ee_rd1 : [~ee_idle] % дожидаемся конца чтения
  ee_rd1 -> wait
  (junction 237) -> (junction 239) [order 2]
  wait -> (junction 237) [order 3] : [sw_ret]
  (junction 239) -> (junction 243) : {temp_ret = false}
  (junction 237) -> (junction 241) [order 1] : [~temp_ret]{temp_ret = true}
  (junction 41) -> (junction 101) [order 2]
  wait -> (junction 41) [order 1] : [sw_rr_stab]
  wait -> (junction 137) [order 2] : [temp_rr]
  (junction 137) -> (junction 22) : [sw_fr_stab]
  (junction 22) -> (junction 107) [order 2]
  (junction 101) -> (junction 43) : {temp_rr = false}
  (junction 41) -> (junction 47) [order 1] : [~temp_rr]{temp_rr = true}
  (junction 22) -> (junction 24) [order 1] : [~temp_fr]{temp_fr = true}
  (junction 107) -> (junction 32) : [temp_fr]{temp_fr = false}
  ee_wr_off -> wait : [~sw_fr_stab && ~sw_rr_stab && ~sw_ret]
  (junction 243) -> (junction 241)
  (junction 43) -> (junction 47)
  (junction 32) -> (junction 24)
  (junction 241) -> (junction 246) : {rele_ret = temp_ret;}
  (junction 47) -> (junction 153) : {rele_rr_stab = temp_rr;
      | rele_fr_stab = temp_fr & temp_rr}
  (junction 24) -> (junction 140) : {rele_fr_stab = temp_fr & temp_rr}
  ee_wr -> ee_wr_off : [~ee_idle] % ждем окончания записи
  ee_idle -> ee_wr : [~res]
  Beep1 -> ee_idle : [i2==0]
  (junction 153) -> (junction 155) [order 1] : [temp_rr]
  (junction 155) -> Beep1 : {i2=1}
  (junction 142) -> Beep1 : {i2=1}
  (junction 140) -> (junction 142) [order 1] : [temp_fr]
  (junction 153) -> (junction 158) [order 2]
  (junction 140) -> (junction 144) [order 2]
  (junction 146) -> Beep1 : {i2=2}
  (junction 144) -> (junction 146)
  (junction 158) -> (junction 160)
  (junction 160) -> Beep1 : {i2=2}
  (junction 246) -> (junction 248) [order 1] : [temp_ret]
  (junction 248) -> Beep1 : {i2=1}
  (junction 246) -> (junction 251) [order 2]
  (junction 251) -> Beep1 : {i2=2}
  data: x function_output; sw_fr_stab input boolean; sw_rr_stab input boolean; rele_fr_stab output =false; rele_rr_stab output =false; i local uint8 =uint8(0); i2 local uint8 =uint8(0); zummer output boolean =false; ee_idle data_store_memory; ee_adr data_store_memory; ee_en_wr data_store_memory; ee_send data_store_memory; ee_en_rd data_store_memory; res local boolean =false; ee_read data_store_memory; adres_stab constant uint8 =uint8(127); temp_fr local boolean; temp_rr local boolean; sw_ret input boolean; rele_ret output boolean; temp_ret local boolean

== stateflow chart BCM2_4/управление страницами и яркостью мониторов/Remote bright ==
  settings: updateMethod=DISCRETE  sampleTime=0.1
  state but_scan [function]
    (default) -> (junction 29)
    (junction 29) -> (junction 30) [order 1] : [inP]{outP=0}
    (junction 29) -> (junction 32) [order 2] : {outP=4}
    (junction 30) -> (junction 34)
    (junction 34) -> (junction 32)
    (junction 32) -> (junction 37)
    (junction 37) -> (junction 39) [order 1] : [inM]{outM=0}
    (junction 37) -> (junction 43) [order 2] : {outM=4}
    (junction 39) -> (junction 41)
    (junction 41) -> (junction 43)
  state scan
    but_scan
  (default) -> scan
  data: outP output uint8 size=1 =uint8(0); inM input boolean size=1; inP input boolean size=1; outM output uint8 size=1 =uint8(0)
